simulink model "Quadcopter_ControllerWithNavigation"  (R2024b)
settings: Solver=FixedStepAuto  StartTime=0.0  StopTime=inf  RelTol=1e-3  EnableMultiTasking=on
undefined symbols (not defined in the file): SampleTime
libraries: px4uORBlib x10, slpidlib x10, simulink x4, uavalgslib x3, px4Utilslib x2, px4Peripheralslib x1, simulink_extras x1, sharedutil x1, sharedtransform x1
(part 1 of 3)
settings Model: ExtModeTrigDuration=10  Creator=The MathWorks, Inc.  LastModifiedBy=davi1
settings SolverCC: PositivePriorityOrder=on  MaxZcPerStep=1
settings OptimizationCC: EnhancedBackFolding=on  PassReuseOutputArgsAs=Individual arguments  ZeroExternalMemoryAtStartup=off  ZeroInternalMemoryAtStartup=off  MaxStackSize=64  OptimizeBlockOrder=speed  DifferentSizesBufferReuse=on  OptimizationCustomize=off  EfficientTunableParamExpr=on
settings DebuggingCC: ParameterTunabilityLossMsg=error
settings HardwareCC: ProdBitPerPointer=32  ProdBitPerSizeT=32  ProdBitPerPtrDiffT=32  ProdLargestAtomicInteger=Long  ProdLargestAtomicFloat=Double  ProdWordSize=32  ProdLongLongMode=on  ProdHWDeviceType=ARM Compatible->ARM Cortex
settings ModelReferenceCC: EnableRefExpFcnMdlSchedulingChecks=on
settings SFSimCC: MATLABDynamicMemAlloc=off  SimTargetLang=C++
settings RTWCC: Description=Embedded Coder  SystemTargetFile=ert.tlc  HardwareBoard=PX4 Pixhawk 6x  TLCOptions="-aInlineSetEventsForThisBaseRateFcn=TLC_FALSE -aSuppressMultiTaskScheduler=TLC_FALSE  -aRateBasedStepFcn=0"  TemplateMakefile=ert_default_tmf  Toolchain=GNU Tools for PX4 Autopilots  TargetLang=C++  GPUComputeCapability=3.5  DLArmComputeVersion=19.05
settings CodeAppCC: ForceParamTrailComments=on  IgnoreCustomStorageClasses=off  MaxIdLength=63  OperatorAnnotations=on  SimulinkDataObjDesc=on  SFDataObjDesc=on  InsertBlockDesc=on
settings ERTTargetCC: ExtModeTransport=3  ExtModeStaticAlloc=on  ExtModeStaticAllocSize=1024  ExtModeMexFile=ext_xcp  ExtModeIntrfLevel=Level2 - Open  InlinedParameterPlacement=Hierarchical

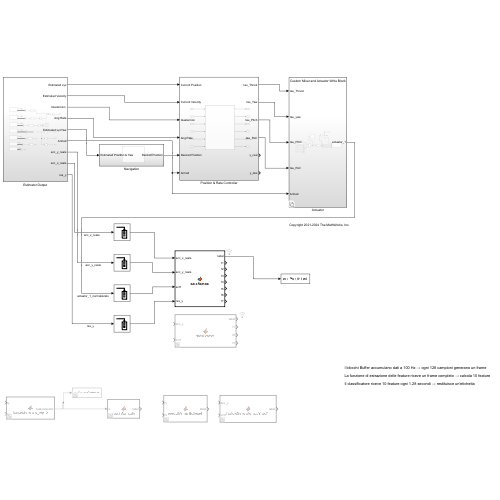
[thumbnail: Simulink's stored preview of the top-level diagram]
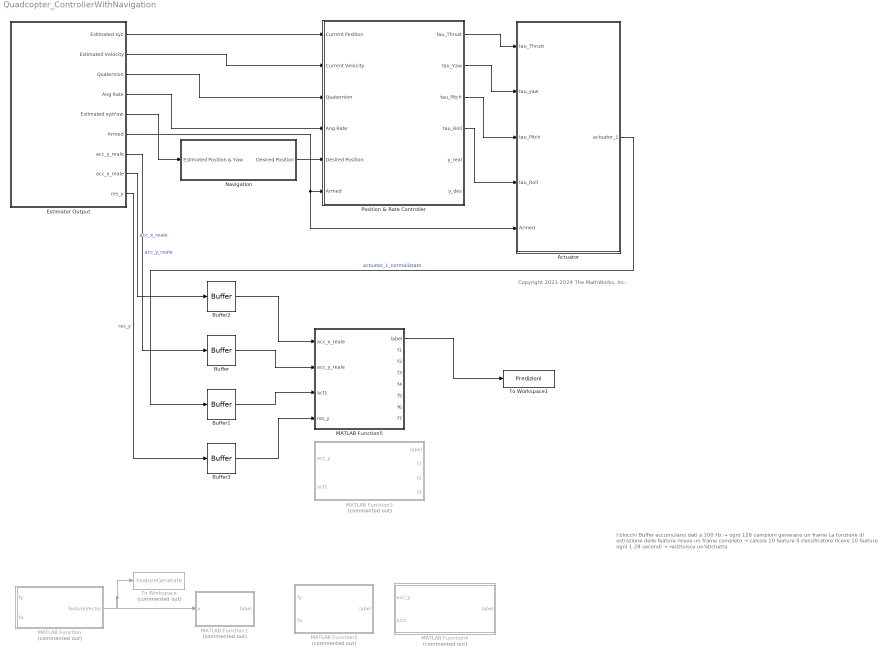
== system Quadcopter_ControllerWithNavigation ==
  note: I blocchi Buffer accumulano dati a 100 Hz → ogni 128 campioni generano un frame
      | La funzione di estrazione delle feature riceve un frame completo → calcola 10 feature
      | Il classificatore riceve 10 feature ogni 1.28 secondi → restituisce un'etichetta
  note: Copyright 2021-2024 The MathWorks, Inc.
  Actuator : Subsystem  Variant=on
  Buffer{,1..3} (4 alike) : Buffer  N=128  V=32  OutputFrames=off
  Estimator Output : Subsystem
  MATLAB Function : MATLAB Function  Commented=on  TreatAsAtomicUnit=on
  MATLAB Function1 : MATLAB Function  Commented=on  TreatAsAtomicUnit=on
  MATLAB Function2 : MATLAB Function  Commented=on  TreatAsAtomicUnit=on
  MATLAB Function3 : MATLAB Function  Commented=on  TreatAsAtomicUnit=on
  MATLAB Function4 : MATLAB Function  Commented=on  TreatAsAtomicUnit=on
  MATLAB Function5 : MATLAB Function  TreatAsAtomicUnit=on
  Navigation : Subsystem
  Position & Rate Controller : Subsystem
  To Workspace : ToWorkspace  Commented=on  VariableName=FeatureGenerate  SampleTime=-1
  To Workspace1 : ToWorkspace  VariableName=Predizioni  SaveFormat=Structure With Time  SampleTime=-1
  wires:
  Estimator Output/1(Estimated xyz) -> Position & Rate Controller/1(Current Position)
  Estimator Output/2(Estimated Velocity) -> Position & Rate Controller/2(Current Velocity)
  Estimator Output/3("Quaternion ") -> Position & Rate Controller/3(Quaternion)
  Navigation/1(Desired Position) -> Position & Rate Controller/5(Desired Position)
  Estimator Output/5(Estimated xyzYaw) -> Navigation/1(Estimated Position & Yaw)
  Estimator Output/4(Ang Rate) -> Position & Rate Controller/4(Ang Rate)
  Estimator Output/6(Armed) -> Actuator/5(Armed), Position & Rate Controller/6(Armed)
  Position & Rate Controller/1(tau_Thrust) -> Actuator/1(tau_Thrust)
  Position & Rate Controller/2(tau_Yaw) -> Actuator/2(tau_yaw)
  Position & Rate Controller/3(tau_Pitch) -> Actuator/3(tau_Pitch)
  Position & Rate Controller/4("tau_Roll ") -> Actuator/4(tau_Roll)
  MATLAB Function/1(featureVector) -> MATLAB Function1/1(x), To Workspace/1
  Estimator Output/7(acc_y_reale) -> Buffer/1  "acc_y_reale"
  Actuator/1(actuator_1) -> Buffer1/1  "actuator_1_normalizzato"
  Estimator Output/8(acc_x_reale) -> Buffer2/1  "acc_x_reale"
  Estimator Output/9(res_y) -> Buffer3/1  "res_y"
  Buffer2/1 -> MATLAB Function5/1(acc_x_reale)
  Buffer3/1 -> MATLAB Function5/4(res_y)
  Buffer/1 -> MATLAB Function5/2(acc_y_reale)
  Buffer1/1 -> MATLAB Function5/3(act1)
  MATLAB Function5/1(label) -> To Workspace1/1

== system Quadcopter_ControllerWithNavigation/Actuator ==
  tau_Thrust : Inport
  tau_yaw : Inport  Port=2
  tau_Pitch : Inport  Port=3
  tau_Roll : Inport  Port=4
  Armed : Inport  Port=5
  Custom Mixer and Actuator Write Block : Subsystem  VariantControl=useCustomMixer == true
  PX4 Mixer and actuator_controls_0 topic : Subsystem  VariantControl=useCustomMixer == false
  actuator_1 : Outport

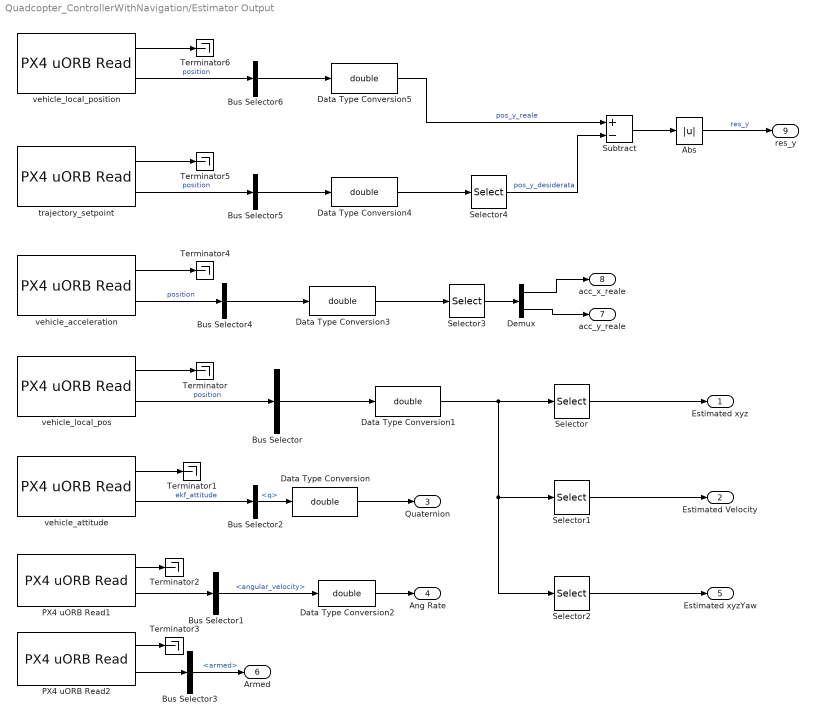
== system Quadcopter_ControllerWithNavigation/Estimator Output ==
  Abs : Abs  SaturateOnIntegerOverflow=off
  Bus Selector : BusSelector  OutputSignals=x,y,z,vx,vy,vz,heading  OutputAsBus=on
  Bus Selector1 : BusSelector  OutputSignals=angular_velocity
  Bus Selector2 : BusSelector  OutputSignals=q
  Bus Selector3 : BusSelector  OutputSignals=armed
  Bus Selector4 : BusSelector  OutputSignals=xyz  OutputAsBus=on
  Bus Selector5 : BusSelector  OutputSignals=position  OutputAsBus=on
  Bus Selector6 : BusSelector  OutputSignals=y  OutputAsBus=on
  Data Type Conversion{,1..5} (6 alike) : DataTypeConversion  OutDataTypeStr=double  SaturateOnIntegerOverflow=off  RndMeth=Floor
  Demux : Demux  Outputs=2
  PX4 uORB Read1 : px4uORBlib/PX4 uORB Read  uORBTopic=VehicleOdometry  selectInstance=vehicle_odometry  SampleTime=-1  BlockingMode=off  BlockTimeout=1e-3
  PX4 uORB Read2 : px4uORBlib/PX4 uORB Read  uORBTopic=ActuatorArmed  selectInstance=ActuatorArmed  SampleTime=-1  BlockingMode=off  BlockTimeout=1e-3
  Selector : Selector  InputPortWidth=7  IndexOptions=Index vector (dialog)  Indices=[1:3]  OutputSizes=1
  Selector1 : Selector  InputPortWidth=7  IndexOptions=Index vector (dialog)  Indices=[4:6]  OutputSizes=1
  Selector2 : Selector  InputPortWidth=7  IndexOptions=Index vector (dialog)  Indices=[1 2 3 7]  OutputSizes=1
  Selector3 : Selector  InputPortWidth=3  IndexOptions=Index vector (dialog)  Indices=[1 2]  OutputSizes=1
  Selector4 : Selector  InputPortWidth=3  IndexOptions=Index vector (dialog)  Indices=[2]  OutputSizes=1
  Subtract : Sum  Inputs=+-
  Terminator{,1..6} (7 alike) : Terminator
  trajectory_setpoint : px4uORBlib/PX4 uORB Read  uORBTopic=TrajectorySetpoint  selectInstance=TrajectorySetpoint  SampleTime=SampleTime  BlockingMode=off  BlockTimeout=1e-3
  vehicle_acceleration : px4uORBlib/PX4 uORB Read  uORBTopic=VehicleAcceleration  selectInstance=VehicleAcceleration  SampleTime=SampleTime  BlockingMode=off  BlockTimeout=1e-3
  vehicle_attitude : px4uORBlib/PX4 uORB Read  uORBTopic=VehicleAttitude  selectInstance=vehicle_attitude  SampleTime=-1  BlockingMode=off  BlockTimeout=1e-3
  vehicle_local_pos : px4uORBlib/PX4 uORB Read  uORBTopic=VehicleLocalPosition  selectInstance=vehicle_local_position  SampleTime=SampleTime  BlockingMode=off  BlockTimeout=1e-3
  vehicle_local_position : px4uORBlib/PX4 uORB Read  uORBTopic=VehicleLocalPosition  selectInstance=vehicle_local_position  SampleTime=SampleTime  BlockingMode=off  BlockTimeout=1e-3
  Estimated xyz : Outport
  Estimated Velocity : Outport  Port=2
  "Quaternion " : Outport  Port=3
  Ang Rate : Outport  Port=4
  Estimated xyzYaw : Outport  Port=5
  Armed : Outport  Port=6
  acc_y_reale : Outport  Port=7
  acc_x_reale : Outport  Port=8
  res_y : Outport  Port=9
  wires:
  Data Type Conversion/1 -> "Quaternion "/1
  Bus Selector2/1 -> Data Type Conversion/1  "<q>"
  vehicle_local_pos/2 -> Bus Selector/1  "position"
  Data Type Conversion1/1 -> Selector1/1, Selector2/1, Selector/1
  Selector2/1 -> Estimated xyzYaw/1
  vehicle_attitude/1 -> Terminator1/1
  vehicle_attitude/2 -> Bus Selector2/1  "ekf_attitude"
  vehicle_local_pos/1 -> Terminator/1
  Selector/1 -> Estimated xyz/1
  Selector1/1 -> Estimated Velocity/1
  Bus Selector/1 -> Data Type Conversion1/1
  PX4 uORB Read1/1 -> Terminator2/1
  Data Type Conversion2/1 -> Ang Rate/1
  PX4 uORB Read1/2 -> Bus Selector1/1
  PX4 uORB Read2/1 -> Terminator3/1
  Bus Selector3/1 -> Armed/1  "<armed>"
  PX4 uORB Read2/2 -> Bus Selector3/1
  Bus Selector1/1 -> Data Type Conversion2/1  "<angular_velocity>"
  vehicle_acceleration/1 -> Terminator4/1
  vehicle_acceleration/2 -> Bus Selector4/1  "position"
  Bus Selector4/1 -> Data Type Conversion3/1
  Data Type Conversion3/1 -> Selector3/1
  Bus Selector5/1 -> Data Type Conversion4/1
  trajectory_setpoint/2 -> Bus Selector5/1  "position"
  trajectory_setpoint/1 -> Terminator5/1
  Data Type Conversion4/1 -> Selector4/1
  Selector3/1 -> Demux/1
  Demux/2 -> acc_y_reale/1
  Demux/1 -> acc_x_reale/1
  vehicle_local_position/1 -> Terminator6/1
  Data Type Conversion5/1 -> Subtract/1  "pos_y_reale"
  vehicle_local_position/2 -> Bus Selector6/1  "position"
  Bus Selector6/1 -> Data Type Conversion5/1
  Selector4/1 -> Subtract/2  "pos_y_desiderata"
  Subtract/1 -> Abs/1
  Abs/1 -> res_y/1  "res_y"

== system Quadcopter_ControllerWithNavigation/Navigation ==
  Estimated Position & Yaw : Inport
  Quadcopter Navigation Algorithm : Subsystem  Variant=on
  Desired Position : Outport
  wires:
  Quadcopter Navigation Algorithm/1(Desired Position) -> Desired Position/1
  Estimated Position & Yaw/1 -> Quadcopter Navigation Algorithm/1(Current Position)

== system Quadcopter_ControllerWithNavigation/Position & Rate Controller ==
  Current Position : Inport
  Current Velocity : Inport  Port=2
  Quaternion : Inport  Port=3
  Ang Rate : Inport  Port=4
  Desired Position : Inport  Port=5
  Armed : Inport  Port=6
  Controller : Subsystem
  tau_Thrust : Outport
  tau_Yaw : Outport  Port=2
  tau_Pitch : Outport  Port=3
  "tau_Roll " : Outport  Port=4
  y_real : Outport  Port=5
  y_des : Outport  Port=6
  wires:
  Controller/3(tau_Pitch) -> tau_Pitch/1
  Quaternion/1 -> Controller/3(Quaternion)
  Controller/2(tau_Yaw) -> tau_Yaw/1
  Controller/4("tau_Roll ") -> "tau_Roll "/1
  Current Velocity/1 -> Controller/2(Velocity)
  Current Position/1 -> Controller/1(Position)
  Controller/1(tau_Thrust) -> tau_Thrust/1
  Desired Position/1 -> Controller/5(Desired Position)
  Ang Rate/1 -> Controller/4(Ang rate)
  Armed/1 -> Controller/6(Armed)
  Controller/5(y_real) -> y_real/1
  Controller/6(y_des) -> y_des/1

== system Quadcopter_ControllerWithNavigation/Actuator/Custom Mixer and Actuator Write Block ==
  tau_Thrust : Inport
  tau_yaw : Inport  Port=2
  tau_Pitch : Inport  Port=3
  tau_Roll : Inport  Port=4
  Armed : Inport  Port=5
  Data Type Conversion : DataTypeConversion  OutDataTypeStr=single  SaturateOnIntegerOverflow=off  RndMeth=Floor
  Demux : Demux
  Display : Display
  Mixer matrix : Constant  Value=[1 1 -1 1;1 -1 1 1;1 1 1 -1;1 -1 -1 -1]  OutDataTypeStr=Inherit: Inherit via back propagation  SampleTime=-1
  Mux1 : Mux
  PX4 Actuator Write : px4Peripheralslib/PX4 Actuator Write  Motor1Enable=on  Motor2Enable=on  Motor3Enable=on  Motor4Enable=on  Motor5Enable=off  Motor6Enable=off  Motor7Enable=off  Motor8Enable=off  Motor9Enable=off  Motor10Enable=off  Motor11Enable=off  Motor12Enable=off  IsMotorArray=off  Servo1Enable=off  Servo2Enable=off  Servo3Enable=off  Servo4Enable=off  Servo5Enable=off  Servo6Enable=off  Servo7Enable=off  Servo8Enable=off  IsServoArray=off
  Product1 : Product  Multiplication=Matrix(*)  RndMeth=Zero
  Saturation : Saturate  UpperLimit=1  LowerLimit=0
  Selector : Selector  InputPortWidth=4  IndexOptions=Index vector (dialog)  Indices=[1]  OutputSizes=1
  To Workspace : ToWorkspace  VariableName=Actuator1  SampleTime=-1
  actuator_1 : Outport
  wires:
  Demux/1 -> PX4 Actuator Write/2
  Demux/2 -> PX4 Actuator Write/3
  Product1/1 -> Display/1, Saturation/1
  Mux1/1 -> Product1/2
  Mixer matrix/1 -> Product1/1
  tau_yaw/1 -> Mux1/4
  tau_Thrust/1 -> Mux1/1  "thrust cmd"
  Saturation/1 -> Data Type Conversion/1
  tau_Roll/1 -> Mux1/3  "roll_cmd"
  Demux/3 -> PX4 Actuator Write/4
  Armed/1 -> PX4 Actuator Write/1
  tau_Pitch/1 -> Mux1/2  "pitch cmd"
  Demux/4 -> PX4 Actuator Write/5
  Data Type Conversion/1 -> Selector/1, Demux/1
  Selector/1 -> To Workspace/1, actuator_1/1

== system Quadcopter_ControllerWithNavigation/Actuator/PX4 Mixer and actuator_controls_0 topic ==
  tau_Thrust : Inport
  tau_yaw : Inport  Port=2
  tau_Pitch : Inport  Port=3
  tau_Roll : Inport  Port=4
  Armed : Inport  Port=5
  Bus Assignment : BusAssignment  AssignedSignals=control
  Constant : Constant  Value=zeros(4,1)
  Data Type Conversion : DataTypeConversion  SaturateOnIntegerOverflow=off  RndMeth=Floor
  Mux : Mux  Inputs=5
  PX4 uORB Message : px4uORBlib/PX4 uORB Message  uORBTopic=actuator_controls  SampleTime=inf  selectInstance=vehicle_gps_position
  PX4 uORB Write : px4uORBlib/PX4 uORB Write  uORBTopic=actuator_controls  selectInstance=actuator_controls_0  MessageQueueLen=1
  Terminator : Terminator
  wires:
  Bus Assignment/1 -> PX4 uORB Write/1
  tau_yaw/1 -> Mux/3
  Data Type Conversion/1 -> Bus Assignment/2
  tau_Roll/1 -> Mux/1  "roll_cmd"
  PX4 uORB Message/1 -> Bus Assignment/1
  Mux/1 -> Data Type Conversion/1
  Constant/1 -> Mux/5
  tau_Pitch/1 -> Mux/2  "pitch cmd"
  tau_Thrust/1 -> Mux/4  "thrust cmd"
  Armed/1 -> Terminator/1

== system Quadcopter_ControllerWithNavigation/Navigation/Quadcopter Navigation Algorithm ==
  Current Position : Inport
  Manual Waypoints : Subsystem  VariantControl=guidanceType == 3
  Manual Waypoints from Simulink Dashboard : Subsystem  VariantControl=guidanceType == 2
  Path Correction from Onboard Computer : Subsystem  VariantControl=guidanceType == 1
  Read waypoint from QGroundControl Mission : Subsystem  VariantControl=guidanceType == 0
  Desired Position : Outport

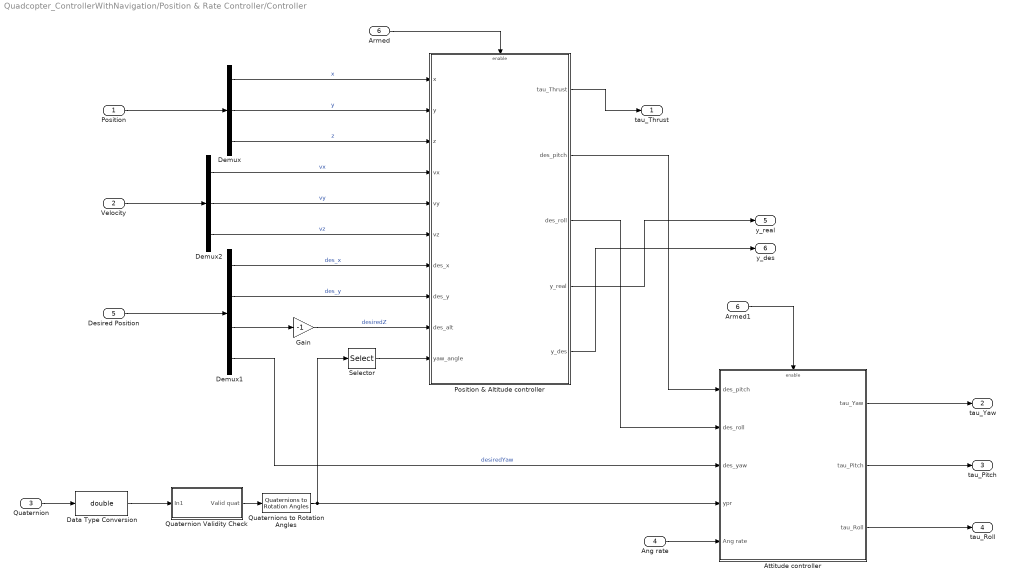
== system Quadcopter_ControllerWithNavigation/Position & Rate Controller/Controller ==
  Position : Inport
  Velocity : Inport  Port=2
  Quaternion : Inport  Port=3
  Ang rate : Inport  Port=4
  Desired Position : Inport  Port=5
  Armed : Inport  Port=6
  Armed1 : InportShadow  Port=6
  Attitude controller : Subsystem
  Data Type Conversion : DataTypeConversion  OutDataTypeStr=double  SaturateOnIntegerOverflow=off  RndMeth=Floor
  Demux : Demux  Outputs=3
  Demux1 : Demux
  Demux2 : Demux  Outputs=3
  Gain : Gain  Gain=-1
  Position & Altitude controller : Subsystem
  Quaternion Validity Check : Subsystem
  Quaternions to Rotation Angles : sharedtransform/Quaternions to Rotation Angles  rotationOrder=ZYX  aMode=aMode
  Selector : Selector  InputPortWidth=3  IndexOptions=Index vector (dialog)  Indices=[1]  OutputSizes=1
  tau_Thrust : Outport
  tau_Yaw : Outport  Port=2
  tau_Pitch : Outport  Port=3
  "tau_Roll " : Outport  Port=4
  y_real : Outport  Port=5
  y_des : Outport  Port=6
  wires:
  Attitude controller/3(tau_Roll) -> "tau_Roll "/1
  Attitude controller/2(tau_Pitch) -> tau_Pitch/1
  Attitude controller/1(tau_Yaw) -> tau_Yaw/1
  Position & Altitude controller/2(des_pitch) -> Attitude controller/1(des_pitch)
  Position & Altitude controller/3(des_roll) -> Attitude controller/2(des_roll)
  Demux/2 -> Position & Altitude controller/2(y)  "y"
  Gain/1 -> Position & Altitude controller/9(des_alt)  "desiredZ"
  Demux2/2 -> Position & Altitude controller/5(vy)  "vy"
  Demux1/1 -> Position & Altitude controller/7(des_x)  "des_x"
  Demux2/1 -> Position & Altitude controller/4(vx)  "vx"
  Demux1/3 -> Gain/1
  Demux/1 -> Position & Altitude controller/1(x)  "x"
  Demux1/2 -> Position & Altitude controller/8(des_y)  "des_y"
  Position & Altitude controller/1(tau_Thrust) -> tau_Thrust/1
  Desired Position/1 -> Demux1/1
  Demux2/3 -> Position & Altitude controller/6(vz)  "vz"
  Demux/3 -> Position & Altitude controller/3(z)  "z"
  Quaternion/1 -> Data Type Conversion/1
  Data Type Conversion/1 -> Quaternion Validity Check/1(In1)
  Position/1 -> Demux/1
  Velocity/1 -> Demux2/1
  Quaternion Validity Check/1(Valid quat) -> Quaternions to Rotation Angles/1
  Ang rate/1 -> Attitude controller/5(Ang rate)
  Quaternions to Rotation Angles/1 -> Selector/1, Attitude controller/4(ypr)
  Selector/1 -> Position & Altitude controller/10(yaw_angle)
  Demux1/4 -> Attitude controller/3(des_yaw)  "desiredYaw"
  Armed/1 -> Position & Altitude controller/Enable
  Armed1/1 -> Attitude controller/Enable
  Position & Altitude controller/4(y_real) -> y_real/1
  Position & Altitude controller/5(y_des) -> y_des/1

== system Quadcopter_ControllerWithNavigation/Navigation/Quadcopter Navigation Algorithm/Manual Waypoints ==
  Current Position : Inport
  Constant1 : Constant  Value=[0 0 -20 0; 20 0 -20 0;20 10 -20 0; 20 100 -30 0;30 100 -30 0;50 100 -30 0]  SampleTime=-1
  Constant2 : Constant  Value=2  SampleTime=-1
  Constant3 : Constant  Value=0  SampleTime=-1
  Mux : Mux  Inputs=2
  Subsystem : Subsystem
  Switch : Switch  Criteria=u2 > Threshold  SaturateOnIntegerOverflow=off  InputSameDT=off
  Terminator1 : Terminator
  Terminator2 : Terminator
  Terminator4 : Terminator
  Waypoint Follower : uavalgslib/Waypoint Follower  UAVType=multirotor  StartFrom=first  TransitionRadiusSource=internal  TransitionRadius=5  MinLookaheadDistance=0.1  HoverAtLastWaypoint=off  YawInput=on  ShowCrossTrackErrorOutput=off  ShowStatusOutput=on  SimulateUsing=Interpreted execution
  Desired Position : Outport
  wires:
  Constant1/1 -> Waypoint Follower/2
  Waypoint Follower/1 -> Subsystem/2(Lookahead Point), Switch/3
  Waypoint Follower/4 -> Terminator4/1
  Subsystem/1(des_landing_pos) -> Switch/1
  Current Position/1 -> Waypoint Follower/1, Subsystem/1(curr_xyzYaw)
  Waypoint Follower/5 -> Switch/2
  Constant2/1 -> Waypoint Follower/3
  Waypoint Follower/2 -> Terminator2/1
  Switch/1 -> Mux/1  "command"
  Mux/1 -> Desired Position/1
  Waypoint Follower/3 -> Terminator1/1
  Constant3/1 -> Mux/2

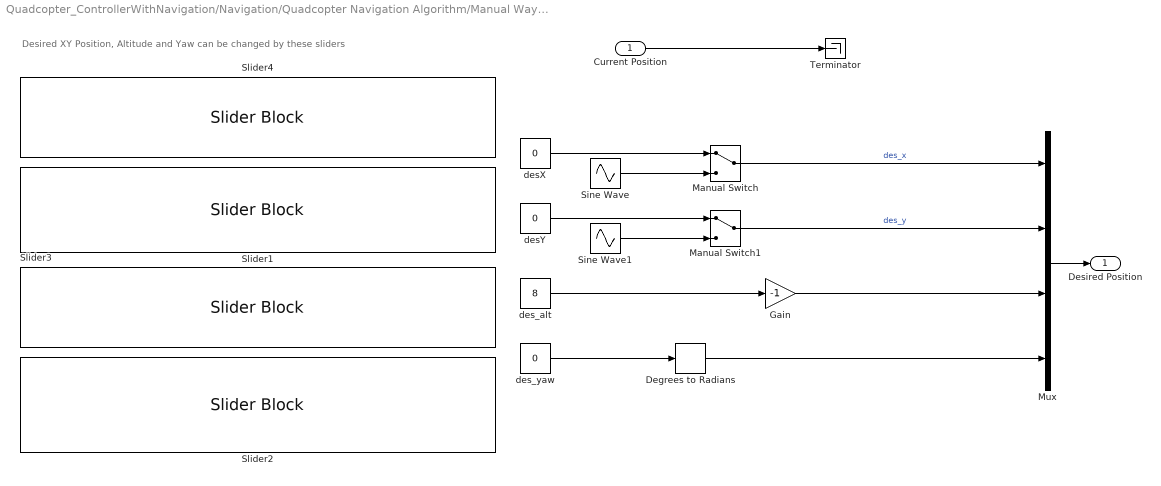
== system Quadcopter_ControllerWithNavigation/Navigation/Quadcopter Navigation Algorithm/Manual Waypoints from Simulink Dashboard ==
  note: Desired XY Position, Altitude and Yaw can be changed by these sliders
  Current Position : Inport  PortDimensions=[1 4]
  Degrees to Radians : simulink_extras/Transformations/Degrees to Radians
  Gain : Gain  Gain=-1
  Manual Switch : ManualSwitch
  Manual Switch1 : ManualSwitch
  Mux : Mux
  Sine Wave : Sin  Amplitude=80  Frequency=2*pi*0.005
  Sine Wave1 : Sin  Amplitude=80  Frequency=2*pi*0.005  Phase=pi/2
  Slider1 : SliderBlock  ScaleMin=-20  ScaleMax=20
  Slider2 : SliderBlock  ScaleMin=-180  ScaleMax=180
  Slider3 : SliderBlock
  Slider4 : SliderBlock  ScaleMin=-20  ScaleMax=20
  Terminator : Terminator
  desX : Constant  Value=0  SampleTime=-1
  desY : Constant  Value=0  SampleTime=-1
  des_alt : Constant  Value=8  SampleTime=-1
  des_yaw : Constant  Value=0  SampleTime=-1
  Desired Position : Outport
  wires:
  des_alt/1 -> Gain/1
  desY/1 -> Manual Switch1/1
  Sine Wave/1 -> Manual Switch/2
  desX/1 -> Manual Switch/1
  Manual Switch1/1 -> Mux/2  "des_y"
  des_yaw/1 -> Degrees to Radians/1
  Manual Switch/1 -> Mux/1  "des_x"
  Sine Wave1/1 -> Manual Switch1/2
  Mux/1 -> Desired Position/1
  Current Position/1 -> Terminator/1
  Gain/1 -> Mux/3
  Degrees to Radians/1 -> Mux/4

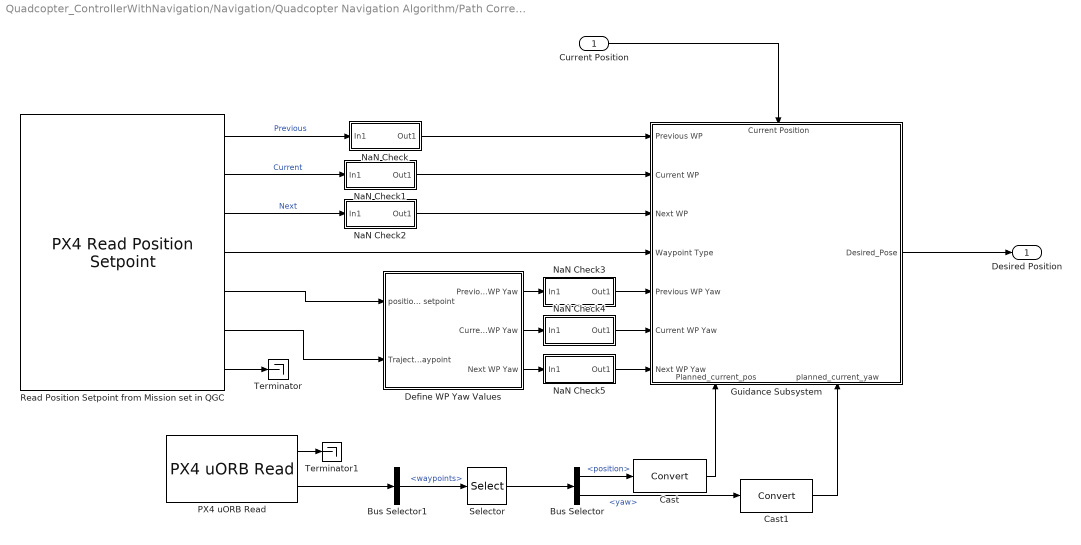
== system Quadcopter_ControllerWithNavigation/Navigation/Quadcopter Navigation Algorithm/Path Correction from Onboard Computer ==
  Current Position : Inport
  Bus Selector : BusSelector  OutputSignals=position,yaw
  Bus Selector1 : BusSelector  OutputSignals=waypoints
  Cast : DataTypeConversion  SaturateOnIntegerOverflow=off  RndMeth=Floor
  Cast1 : DataTypeConversion  SaturateOnIntegerOverflow=off  RndMeth=Floor
  "Define WP Yaw Values " : Subsystem
  Guidance Subsystem : Subsystem
      settings: PortSchema="{\"entries\":[{\"content\":{\"sides\":[{\"content\":{\"connectorIds\":[\"In1\",\"In2\",\"In3\",\"In4\",\"In5\",\"In6\",\"In7\"]},\"type\":\"ConnectorPlacement.EquallySpacedRectSide\",\"uuid\":\"e9e96be5-af21-4911-860e-f3d41d3d51a5\"},{\"content\":{\"connectorIds\":[\"Out1\"],\"side\":\"RIGHT\"},\"type\":\"ConnectorPlacement.EquallySpacedRectSide\",\"uuid\":\"1d190cc4-2348-4eca-a529-c9f1d728b718\"},{\"content\":{\"connectorIds\":[\"In8\"],\"side\":\"TOP\"},\"type\":\"ConnectorPlacement.EquallySpacedRectSide\",\"uuid\":\"c248d3d5-3b30-416c-a277-519f6ee966ff\"},{\"content\":{\"connectorIds\":[\"In9\",\"In10\"],\"side\":\"BOTTOM\"},\"type\":\"ConnectorPlacement.EquallySpacedRectSide\",\"uuid\":\"2b8da87f-17bd-449d-af9e-128c1548c7b5\"}]},\"type\":\"ConnectorPlacement.EquallySpacedConnector\",\"uuid\":\"bbf0c511-85fc-440a-b356-10e645af4727\"}],\"packageUris\":[\"http://schema.mathworks.com/mf0/Connector/R2020b\"],\"version\":\"1.0\"}"
  NaN Check : Subsystem
  NaN Check1 : Subsystem
  NaN Check2 : Subsystem
  NaN Check3 : Subsystem
  NaN Check4 : Subsystem
  NaN Check5 : Subsystem
  PX4 uORB Read : px4uORBlib/PX4 uORB Read  uORBTopic=vehicle_trajectory_waypoint  selectInstance=vehicle_trajectory_waypoint_desired  SampleTime=SampleTime  BlockingMode=off  BlockTimeout=1e-3
  Read Position Setpoint from Mission set in QGC : px4Utilslib/PX4 Read Position Setpoint  coordinateFrame=Local Coordinates (NED)  SampleTime=SampleTime  positionSetpointBus=on  trajectoryWaypointsBus=on  onboardFailsafeFlag=off  onboardEnableStatus=on
  Selector : Selector  InputPortWidth=5  IndexOptions=Index vector (dialog)  Indices=2  OutputSizes=1
  Terminator : Terminator
  Terminator1 : Terminator
  Desired Position : Outport
  wires:
  Read Position Setpoint from Mission set in QGC/2 -> NaN Check1/1(In1)  "Current"
  Read Position Setpoint from Mission set in QGC/4 -> Guidance Subsystem/4(Waypoint Type)
  Read Position Setpoint from Mission set in QGC/1 -> NaN Check/1(In1)  "Previous"
  Guidance Subsystem/1(Desired_Pose) -> Desired Position/1
  Read Position Setpoint from Mission set in QGC/3 -> NaN Check2/1(In1)  "Next"
  Current Position/1 -> Guidance Subsystem/8(Current Position)
  Read Position Setpoint from Mission set in QGC/7 -> Terminator/1
  Read Position Setpoint from Mission set in QGC/6 -> "Define WP Yaw Values "/2(Trajectory Waypoint)
  Read Position Setpoint from Mission set in QGC/5 -> "Define WP Yaw Values "/1(position setpoint)
  "Define WP Yaw Values "/3(Next WP Yaw) -> NaN Check5/1(In1)
  "Define WP Yaw Values "/2(Current WP Yaw) -> NaN Check4/1(In1)
  "Define WP Yaw Values "/1(Previous WP Yaw) -> NaN Check3/1(In1)
  PX4 uORB Read/1 -> Terminator1/1
  Bus Selector/1 -> Cast/1  "<position>"
  PX4 uORB Read/2 -> Bus Selector1/1
  Selector/1 -> Bus Selector/1
  Bus Selector/2 -> Cast1/1  "<yaw>"
  Bus Selector1/1 -> Selector/1  "<waypoints>"
  Cast/1 -> Guidance Subsystem/9(Planned_current_pos)
  Cast1/1 -> Guidance Subsystem/10(planned_current_yaw)
  NaN Check/1(Out1) -> Guidance Subsystem/1(Previous WP)
  NaN Check1/1(Out1) -> Guidance Subsystem/2(Current WP)
  NaN Check2/1(Out1) -> Guidance Subsystem/3(Next WP)
  NaN Check3/1(Out1) -> Guidance Subsystem/5(Previous WP Yaw)
  NaN Check4/1(Out1) -> Guidance Subsystem/6(Current WP Yaw)
  NaN Check5/1(Out1) -> Guidance Subsystem/7(Next WP Yaw)

== system Quadcopter_ControllerWithNavigation/Navigation/Quadcopter Navigation Algorithm/Read waypoint from QGroundControl Mission ==
  Current Position : Inport
  Guidance Subsystem : Subsystem
      settings: PortSchema="{\"entries\":[{\"content\":{\"sides\":[{\"content\":{\"connectorIds\":[\"In1\",\"In2\",\"In3\",\"In4\"]},\"type\":\"ConnectorPlacement.EquallySpacedRectSide\",\"uuid\":\"e9e96be5-af21-4911-860e-f3d41d3d51a5\"},{\"content\":{\"connectorIds\":[\"Out1\"],\"side\":\"RIGHT\"},\"type\":\"ConnectorPlacement.EquallySpacedRectSide\",\"uuid\":\"1d190cc4-2348-4eca-a529-c9f1d728b718\"},{\"content\":{\"connectorIds\":[\"In5\"],\"side\":\"TOP\"},\"type\":\"ConnectorPlacement.EquallySpacedRectSide\",\"uuid\":\"c248d3d5-3b30-416c-a277-519f6ee966ff\"}]},\"type\":\"ConnectorPlacement.EquallySpacedConnector\",\"uuid\":\"bbf0c511-85fc-440a-b356-10e645af4727\"}],\"packageUris\":[\"http://schema.mathworks.com/mf0/Connector/R2020b\"],\"version\":\"1.0\"}"
  Read Position Setpoint from Mission set in QGC : px4Utilslib/PX4 Read Position Setpoint  coordinateFrame=Local Coordinates (NED)  SampleTime=SampleTime  positionSetpointBus=off  trajectoryWaypointsBus=off  onboardFailsafeFlag=off  onboardEnableStatus=off
  Desired Position : Outport
  wires:
  Read Position Setpoint from Mission set in QGC/1 -> Guidance Subsystem/1(Previous WP)  "Previous"
  Read Position Setpoint from Mission set in QGC/4 -> Guidance Subsystem/4(Waypoint Type)
  Read Position Setpoint from Mission set in QGC/2 -> Guidance Subsystem/2(Current WP)  "Current"
  Guidance Subsystem/1(Desired_Pose) -> Desired Position/1
  Read Position Setpoint from Mission set in QGC/3 -> Guidance Subsystem/3(Next WP)  "Next"
  Current Position/1 -> Guidance Subsystem/5(Current Position)

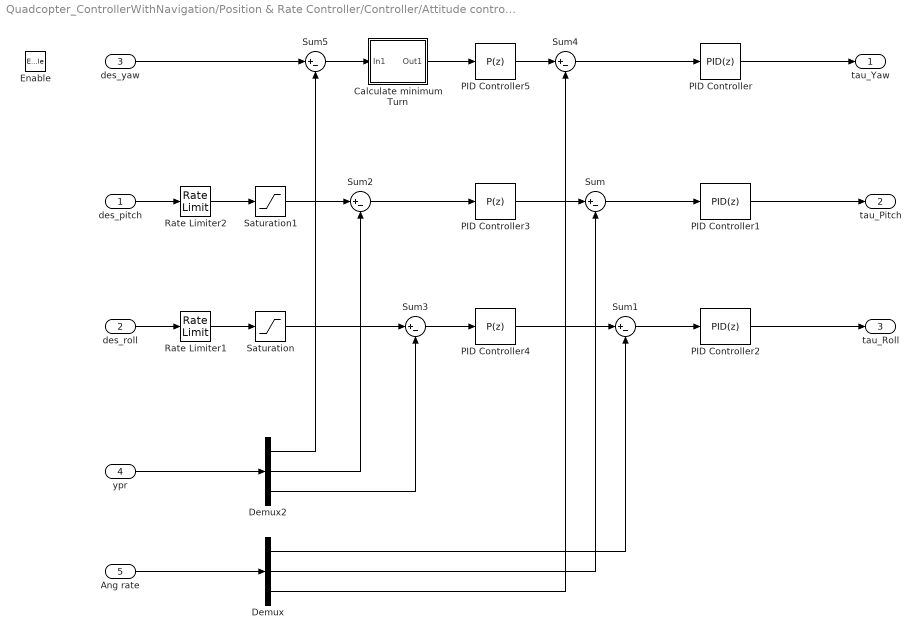
== system Quadcopter_ControllerWithNavigation/Position & Rate Controller/Controller/Attitude controller ==
  des_pitch : Inport
  des_roll : Inport  Port=2
  des_yaw : Inport  Port=3
  ypr : Inport  Port=4
  Ang rate : Inport  Port=5
  Enable : EnablePort
  Calculate minimum Turn : Subsystem
  Demux : Demux  Outputs=3
  Demux2 : Demux  Outputs=3
  PID Controller : slpidlib/PID Controller  Controller=PID  Form=Parallel  TimeDomain=Discrete-time  UseExternalTs=off  SampleTime=-1  IntegratorMethod=Forward Euler  FilterMethod=Forward Euler  ControllerParametersSource=internal  P=0.2  I=0  UseKiTs=off  D=0  UseExternalDerivativeSource=off  N=100  UseFilter=on  TunerSelectOption=Transfer Function Based (PID Tuner App)  InitialConditionSource=internal  InitialConditionForIntegrator=0  InitialConditionForFilter=0  DifferentiatorICPrevScaledInput=0  ExternalReset=none  TrackingMode=off  Kt=1  LimitOutput=on  SatLimitsSource=internal  UpperSaturationLimit=0.1  LowerSaturationLimit=-0.1  LinearizeAsGain=on  AntiWindupMode=clamping  Kb=1  LimitIntegrator=off  UpperIntegratorSaturationLimit=inf  LowerIntegratorSaturationLimit=-inf  POutMin=[]  POutMax=[]  IOutMin=[]  IOutMax=[]  DOutMin=[]  DOutMax=[]  NOutMin=[]  NOutMax=[]  SumOutMin=[]  SumOutMax=[]  SaturationOutMin=[]  SaturationOutMax=[]  PParamMin=[]  PParamMax=[]  IParamMin=[]  IParamMax=[]  DParamMin=[]  DParamMax=[]  NParamMin=[]  NParamMax=[]  KbParamMin=[]  KbParamMax=[]  KtParamMin=[]  KtParamMax=[]  KbOutMin=[]  KbOutMax=[]  KtOutMin=[]  KtOutMax=[]  IntegratorOutMin=[]  IntegratorOutMax=[]  FilterOutMin=[]  FilterOutMax=[]  SumI1OutMin=[]  SumI1OutMax=[]  SumI2OutMin=[]  SumI2OutMax=[]  SumI3OutMin=[]  SumI3OutMax=[]  SumI4OutMin=[]  SumI4OutMax=[]  SumDOutMin=[]  SumDOutMax=[]  DifferentiatorOutMin=[]  DifferentiatorOutMax=[]  FilterDiffOutCoefMin=[]  FilterDiffOutCoefMax=[]  ReciprocalOutMin=[]  ReciprocalOutMax=[]  SumDenOutMin=[]  SumDenOutMax=[]  SumNumOutMin=[]  SumNumOutMax=[]  DivideOutMin=[]  DivideOutMax=[]  UdiffTsProdOutMin=[]  UdiffTsProdOutMax=[]  NTsProdOutMin=[]  NTsProdOutMax=[]  UintegralTsProdOutMin=[]  UintegralTsProdOutMax=[]  UngainTsProdOutMin=[]  UngainTsProdOutMax=[]  ClampingZeroOutDataTypeStr=Inherit: Inherit via back propagation  ClampingZeroOutMin=[]  ClampingZeroOutMax=[]  FilterDenConstantOutDataTypeStr=Inherit: Inherit via back propagation  FilterDenConstantOutMin=[]  FilterDenConstantOutMax=[]  PCopyOutDataTypeStr=Inherit: Inherit via back propagation  PCopyOutMin=[]  PCopyOutMax=[]  NCopyOutDataTypeStr=Inherit: Inherit via back propagation  NCopyOutMin=[]  NCopyOutMax=[]  IntegratorContinuousStateAttributes=''  IntegratorStateMustResolveToSignalObject=off  IntegratorRTWStateStorageClass=Auto  FilterContinuousStateAttributes=''  FilterStateMustResolveToSignalObject=off  FilterRTWStateStorageClass=Auto  ParallelPVariant=InternalParameters  IdealPVariant=Disabled  IVariant=InternalParameters  DVariant=InternalParameters  IntegratorVariant=Discrete  SatVariant=Enabled  AWVariant=DiscClampingParallel  PCopyVariant=Disabled  TRVariant=Disabled  FdbkBlocksVariant=Forward  IdealPFdbkVariant=Disabled  SatFdbkVariant=Disabled  DerivativeFilterVariant=ForwardEulerFilter  NVariant=InternalParameters  NCopyVariant=Disabled  FilterICVariant=InternalICsFilter  IntegratorICVariant=InternalICs  ExternalResetVariant=Disabled  TRSumVariant=Passthrough  SumFdbkVariant=Disabled  SumVariant=Sum_PID  TsampFilterVariant=InternalTs  TsampNgainVariant=Passthrough  TsampIntegralVariant=Disabled_SignalSpec  ExternalSaturationOutDataTypeStr=Inherit: Same as second input  DerivativeSourceVariant=ErrorSignal  PreIntVariant=InternalPreInt
  PID Controller1 : slpidlib/PID Controller  Controller=PID  Form=Parallel  TimeDomain=Discrete-time  UseExternalTs=off  SampleTime=-1  IntegratorMethod=Forward Euler  FilterMethod=Forward Euler  ControllerParametersSource=internal  P=0.035  I=0  UseKiTs=off  D=0.05/20  UseExternalDerivativeSource=off  N=50  UseFilter=on  TunerSelectOption=Transfer Function Based (PID Tuner App)  InitialConditionSource=internal  InitialConditionForIntegrator=0  InitialConditionForFilter=0  DifferentiatorICPrevScaledInput=0  ExternalReset=none  TrackingMode=off  Kt=1  LimitOutput=on  SatLimitsSource=internal  UpperSaturationLimit=0.2  LowerSaturationLimit=-0.2  LinearizeAsGain=on  AntiWindupMode=clamping  Kb=1  LimitIntegrator=off  UpperIntegratorSaturationLimit=inf  LowerIntegratorSaturationLimit=-inf  POutMin=[]  POutMax=[]  IOutMin=[]  IOutMax=[]  DOutMin=[]  DOutMax=[]  NOutMin=[]  NOutMax=[]  SumOutMin=[]  SumOutMax=[]  SaturationOutMin=[]  SaturationOutMax=[]  PParamMin=[]  PParamMax=[]  IParamMin=[]  IParamMax=[]  DParamMin=[]  DParamMax=[]  NParamMin=[]  NParamMax=[]  KbParamMin=[]  KbParamMax=[]  KtParamMin=[]  KtParamMax=[]  KbOutMin=[]  KbOutMax=[]  KtOutMin=[]  KtOutMax=[]  IntegratorOutMin=[]  IntegratorOutMax=[]  FilterOutMin=[]  FilterOutMax=[]  SumI1OutMin=[]  SumI1OutMax=[]  SumI2OutMin=[]  SumI2OutMax=[]  SumI3OutMin=[]  SumI3OutMax=[]  SumI4OutMin=[]  SumI4OutMax=[]  SumDOutMin=[]  SumDOutMax=[]  DifferentiatorOutMin=[]  DifferentiatorOutMax=[]  FilterDiffOutCoefMin=[]  FilterDiffOutCoefMax=[]  ReciprocalOutMin=[]  ReciprocalOutMax=[]  SumDenOutMin=[]  SumDenOutMax=[]  SumNumOutMin=[]  SumNumOutMax=[]  DivideOutMin=[]  DivideOutMax=[]  UdiffTsProdOutMin=[]  UdiffTsProdOutMax=[]  NTsProdOutMin=[]  NTsProdOutMax=[]  UintegralTsProdOutMin=[]  UintegralTsProdOutMax=[]  UngainTsProdOutMin=[]  UngainTsProdOutMax=[]  ClampingZeroOutDataTypeStr=Inherit: Inherit via back propagation  ClampingZeroOutMin=[]  ClampingZeroOutMax=[]  FilterDenConstantOutDataTypeStr=Inherit: Inherit via back propagation  FilterDenConstantOutMin=[]  FilterDenConstantOutMax=[]  PCopyOutDataTypeStr=Inherit: Inherit via back propagation  PCopyOutMin=[]  PCopyOutMax=[]  NCopyOutDataTypeStr=Inherit: Inherit via back propagation  NCopyOutMin=[]  NCopyOutMax=[]  IntegratorContinuousStateAttributes=''  IntegratorStateMustResolveToSignalObject=off  IntegratorRTWStateStorageClass=Auto  FilterContinuousStateAttributes=''  FilterStateMustResolveToSignalObject=off  FilterRTWStateStorageClass=Auto  ParallelPVariant=InternalParameters  IdealPVariant=Disabled  IVariant=InternalParameters  DVariant=InternalParameters  IntegratorVariant=Discrete  SatVariant=Enabled  AWVariant=DiscClampingParallel  PCopyVariant=Disabled  TRVariant=Disabled  FdbkBlocksVariant=Forward  IdealPFdbkVariant=Disabled  SatFdbkVariant=Disabled  DerivativeFilterVariant=ForwardEulerFilter  NVariant=InternalParameters  NCopyVariant=Disabled  FilterICVariant=InternalICsFilter  IntegratorICVariant=InternalICs  ExternalResetVariant=Disabled  TRSumVariant=Passthrough  SumFdbkVariant=Disabled  SumVariant=Sum_PID  TsampFilterVariant=InternalTs  TsampNgainVariant=Passthrough  TsampIntegralVariant=Disabled_SignalSpec  ExternalSaturationOutDataTypeStr=Inherit: Same as second input  DerivativeSourceVariant=ErrorSignal  PreIntVariant=InternalPreInt
  PID Controller2 : slpidlib/PID Controller  Controller=PID  Form=Parallel  TimeDomain=Discrete-time  UseExternalTs=off  SampleTime=-1  IntegratorMethod=Forward Euler  FilterMethod=Forward Euler  ControllerParametersSource=internal  P=0.035  I=0  UseKiTs=off  D=0.05/20  UseExternalDerivativeSource=off  N=50  UseFilter=on  TunerSelectOption=Transfer Function Based (PID Tuner App)  InitialConditionSource=internal  InitialConditionForIntegrator=0  InitialConditionForFilter=0  DifferentiatorICPrevScaledInput=0  ExternalReset=none  TrackingMode=off  Kt=1  LimitOutput=on  SatLimitsSource=internal  UpperSaturationLimit=0.2  LowerSaturationLimit=-0.2  LinearizeAsGain=on  AntiWindupMode=clamping  Kb=1  LimitIntegrator=off  UpperIntegratorSaturationLimit=inf  LowerIntegratorSaturationLimit=-inf  POutMin=[]  POutMax=[]  IOutMin=[]  IOutMax=[]  DOutMin=[]  DOutMax=[]  NOutMin=[]  NOutMax=[]  SumOutMin=[]  SumOutMax=[]  SaturationOutMin=[]  SaturationOutMax=[]  PParamMin=[]  PParamMax=[]  IParamMin=[]  IParamMax=[]  DParamMin=[]  DParamMax=[]  NParamMin=[]  NParamMax=[]  KbParamMin=[]  KbParamMax=[]  KtParamMin=[]  KtParamMax=[]  KbOutMin=[]  KbOutMax=[]  KtOutMin=[]  KtOutMax=[]  IntegratorOutMin=[]  IntegratorOutMax=[]  FilterOutMin=[]  FilterOutMax=[]  SumI1OutMin=[]  SumI1OutMax=[]  SumI2OutMin=[]  SumI2OutMax=[]  SumI3OutMin=[]  SumI3OutMax=[]  SumI4OutMin=[]  SumI4OutMax=[]  SumDOutMin=[]  SumDOutMax=[]  DifferentiatorOutMin=[]  DifferentiatorOutMax=[]  FilterDiffOutCoefMin=[]  FilterDiffOutCoefMax=[]  ReciprocalOutMin=[]  ReciprocalOutMax=[]  SumDenOutMin=[]  SumDenOutMax=[]  SumNumOutMin=[]  SumNumOutMax=[]  DivideOutMin=[]  DivideOutMax=[]  UdiffTsProdOutMin=[]  UdiffTsProdOutMax=[]  NTsProdOutMin=[]  NTsProdOutMax=[]  UintegralTsProdOutMin=[]  UintegralTsProdOutMax=[]  UngainTsProdOutMin=[]  UngainTsProdOutMax=[]  ClampingZeroOutDataTypeStr=Inherit: Inherit via back propagation  ClampingZeroOutMin=[]  ClampingZeroOutMax=[]  FilterDenConstantOutDataTypeStr=Inherit: Inherit via back propagation  FilterDenConstantOutMin=[]  FilterDenConstantOutMax=[]  PCopyOutDataTypeStr=Inherit: Inherit via back propagation  PCopyOutMin=[]  PCopyOutMax=[]  NCopyOutDataTypeStr=Inherit: Inherit via back propagation  NCopyOutMin=[]  NCopyOutMax=[]  IntegratorContinuousStateAttributes=''  IntegratorStateMustResolveToSignalObject=off  IntegratorRTWStateStorageClass=Auto  FilterContinuousStateAttributes=''  FilterStateMustResolveToSignalObject=off  FilterRTWStateStorageClass=Auto  ParallelPVariant=InternalParameters  IdealPVariant=Disabled  IVariant=InternalParameters  DVariant=InternalParameters  IntegratorVariant=Discrete  SatVariant=Enabled  AWVariant=DiscClampingParallel  PCopyVariant=Disabled  TRVariant=Disabled  FdbkBlocksVariant=Forward  IdealPFdbkVariant=Disabled  SatFdbkVariant=Disabled  DerivativeFilterVariant=ForwardEulerFilter  NVariant=InternalParameters  NCopyVariant=Disabled  FilterICVariant=InternalICsFilter  IntegratorICVariant=InternalICs  ExternalResetVariant=Disabled  TRSumVariant=Passthrough  SumFdbkVariant=Disabled  SumVariant=Sum_PID  TsampFilterVariant=InternalTs  TsampNgainVariant=Passthrough  TsampIntegralVariant=Disabled_SignalSpec  ExternalSaturationOutDataTypeStr=Inherit: Same as second input  DerivativeSourceVariant=ErrorSignal  PreIntVariant=InternalPreInt
  PID Controller3 : slpidlib/PID Controller  Controller=P  Form=Parallel  TimeDomain=Discrete-time  UseExternalTs=off  SampleTime=-1  IntegratorMethod=Forward Euler  FilterMethod=Forward Euler  ControllerParametersSource=internal  P=4  I=1  UseKiTs=off  D=0  UseExternalDerivativeSource=off  N=100  UseFilter=on  TunerSelectOption=Transfer Function Based (PID Tuner App)  InitialConditionSource=internal  InitialConditionForIntegrator=0  InitialConditionForFilter=0  DifferentiatorICPrevScaledInput=0  ExternalReset=none  TrackingMode=off  Kt=1  LimitOutput=off  SatLimitsSource=internal  UpperSaturationLimit=inf  LowerSaturationLimit=-inf  LinearizeAsGain=on  AntiWindupMode=none  Kb=1  LimitIntegrator=off  UpperIntegratorSaturationLimit=inf  LowerIntegratorSaturationLimit=-inf  POutMin=[]  POutMax=[]  IOutMin=[]  IOutMax=[]  DOutMin=[]  DOutMax=[]  NOutMin=[]  NOutMax=[]  SumOutMin=[]  SumOutMax=[]  SaturationOutMin=[]  SaturationOutMax=[]  PParamMin=[]  PParamMax=[]  IParamMin=[]  IParamMax=[]  DParamMin=[]  DParamMax=[]  NParamMin=[]  NParamMax=[]  KbParamMin=[]  KbParamMax=[]  KtParamMin=[]  KtParamMax=[]  KbOutMin=[]  KbOutMax=[]  KtOutMin=[]  KtOutMax=[]  IntegratorOutMin=[]  IntegratorOutMax=[]  FilterOutMin=[]  FilterOutMax=[]  SumI1OutMin=[]  SumI1OutMax=[]  SumI2OutMin=[]  SumI2OutMax=[]  SumI3OutMin=[]  SumI3OutMax=[]  SumI4OutMin=[]  SumI4OutMax=[]  SumDOutMin=[]  SumDOutMax=[]  DifferentiatorOutMin=[]  DifferentiatorOutMax=[]  FilterDiffOutCoefMin=[]  FilterDiffOutCoefMax=[]  ReciprocalOutMin=[]  ReciprocalOutMax=[]  SumDenOutMin=[]  SumDenOutMax=[]  SumNumOutMin=[]  SumNumOutMax=[]  DivideOutMin=[]  DivideOutMax=[]  UdiffTsProdOutMin=[]  UdiffTsProdOutMax=[]  NTsProdOutMin=[]  NTsProdOutMax=[]  UintegralTsProdOutMin=[]  UintegralTsProdOutMax=[]  UngainTsProdOutMin=[]  UngainTsProdOutMax=[]  ClampingZeroOutDataTypeStr=Inherit: Inherit via back propagation  ClampingZeroOutMin=[]  ClampingZeroOutMax=[]  FilterDenConstantOutDataTypeStr=Inherit: Inherit via back propagation  FilterDenConstantOutMin=[]  FilterDenConstantOutMax=[]  PCopyOutDataTypeStr=Inherit: Inherit via back propagation  PCopyOutMin=[]  PCopyOutMax=[]  NCopyOutDataTypeStr=Inherit: Inherit via back propagation  NCopyOutMin=[]  NCopyOutMax=[]  IntegratorContinuousStateAttributes=''  IntegratorStateMustResolveToSignalObject=off  IntegratorRTWStateStorageClass=Auto  FilterContinuousStateAttributes=''  FilterStateMustResolveToSignalObject=off  FilterRTWStateStorageClass=Auto  ParallelPVariant=InternalParameters  IdealPVariant=Disabled  IVariant=Disabled  DVariant=Disabled  IntegratorVariant=Disabled  SatVariant=Disabled  AWVariant=Disabled  PCopyVariant=Disabled  TRVariant=Disabled  FdbkBlocksVariant=Forward  IdealPFdbkVariant=Disabled  SatFdbkVariant=Disabled  DerivativeFilterVariant=Disabled  NVariant=Disabled  NCopyVariant=Disabled_SignalSpec  FilterICVariant=Disabled  IntegratorICVariant=Disabled  ExternalResetVariant=Disabled  TRSumVariant=Passthrough  SumFdbkVariant=Disabled  SumVariant=Passthrough_P  TsampFilterVariant=InternalTs  TsampNgainVariant=Passthrough  TsampIntegralVariant=Disabled_SignalSpec  ExternalSaturationOutDataTypeStr=Inherit: Same as second input  DerivativeSourceVariant=Disabled  PreIntVariant=InternalPreInt
  PID Controller4 : slpidlib/PID Controller  Controller=P  Form=Parallel  TimeDomain=Discrete-time  UseExternalTs=off  SampleTime=-1  IntegratorMethod=Forward Euler  FilterMethod=Forward Euler  ControllerParametersSource=internal  P=4  I=1  UseKiTs=off  D=0  UseExternalDerivativeSource=off  N=100  UseFilter=on  TunerSelectOption=Transfer Function Based (PID Tuner App)  InitialConditionSource=internal  InitialConditionForIntegrator=0  InitialConditionForFilter=0  DifferentiatorICPrevScaledInput=0  ExternalReset=none  TrackingMode=off  Kt=1  LimitOutput=off  SatLimitsSource=internal  UpperSaturationLimit=inf  LowerSaturationLimit=-inf  LinearizeAsGain=on  AntiWindupMode=none  Kb=1  LimitIntegrator=off  UpperIntegratorSaturationLimit=inf  LowerIntegratorSaturationLimit=-inf  POutMin=[]  POutMax=[]  IOutMin=[]  IOutMax=[]  DOutMin=[]  DOutMax=[]  NOutMin=[]  NOutMax=[]  SumOutMin=[]  SumOutMax=[]  SaturationOutMin=[]  SaturationOutMax=[]  PParamMin=[]  PParamMax=[]  IParamMin=[]  IParamMax=[]  DParamMin=[]  DParamMax=[]  NParamMin=[]  NParamMax=[]  KbParamMin=[]  KbParamMax=[]  KtParamMin=[]  KtParamMax=[]  KbOutMin=[]  KbOutMax=[]  KtOutMin=[]  KtOutMax=[]  IntegratorOutMin=[]  IntegratorOutMax=[]  FilterOutMin=[]  FilterOutMax=[]  SumI1OutMin=[]  SumI1OutMax=[]  SumI2OutMin=[]  SumI2OutMax=[]  SumI3OutMin=[]  SumI3OutMax=[]  SumI4OutMin=[]  SumI4OutMax=[]  SumDOutMin=[]  SumDOutMax=[]  DifferentiatorOutMin=[]  DifferentiatorOutMax=[]  FilterDiffOutCoefMin=[]  FilterDiffOutCoefMax=[]  ReciprocalOutMin=[]  ReciprocalOutMax=[]  SumDenOutMin=[]  SumDenOutMax=[]  SumNumOutMin=[]  SumNumOutMax=[]  DivideOutMin=[]  DivideOutMax=[]  UdiffTsProdOutMin=[]  UdiffTsProdOutMax=[]  NTsProdOutMin=[]  NTsProdOutMax=[]  UintegralTsProdOutMin=[]  UintegralTsProdOutMax=[]  UngainTsProdOutMin=[]  UngainTsProdOutMax=[]  ClampingZeroOutDataTypeStr=Inherit: Inherit via back propagation  ClampingZeroOutMin=[]  ClampingZeroOutMax=[]  FilterDenConstantOutDataTypeStr=Inherit: Inherit via back propagation  FilterDenConstantOutMin=[]  FilterDenConstantOutMax=[]  PCopyOutDataTypeStr=Inherit: Inherit via back propagation  PCopyOutMin=[]  PCopyOutMax=[]  NCopyOutDataTypeStr=Inherit: Inherit via back propagation  NCopyOutMin=[]  NCopyOutMax=[]  IntegratorContinuousStateAttributes=''  IntegratorStateMustResolveToSignalObject=off  IntegratorRTWStateStorageClass=Auto  FilterContinuousStateAttributes=''  FilterStateMustResolveToSignalObject=off  FilterRTWStateStorageClass=Auto  ParallelPVariant=InternalParameters  IdealPVariant=Disabled  IVariant=Disabled  DVariant=Disabled  IntegratorVariant=Disabled  SatVariant=Disabled  AWVariant=Disabled  PCopyVariant=Disabled  TRVariant=Disabled  FdbkBlocksVariant=Forward  IdealPFdbkVariant=Disabled  SatFdbkVariant=Disabled  DerivativeFilterVariant=Disabled  NVariant=Disabled  NCopyVariant=Disabled_SignalSpec  FilterICVariant=Disabled  IntegratorICVariant=Disabled  ExternalResetVariant=Disabled  TRSumVariant=Passthrough  SumFdbkVariant=Disabled  SumVariant=Passthrough_P  TsampFilterVariant=InternalTs  TsampNgainVariant=Passthrough  TsampIntegralVariant=Disabled_SignalSpec  ExternalSaturationOutDataTypeStr=Inherit: Same as second input  DerivativeSourceVariant=Disabled  PreIntVariant=InternalPreInt
  PID Controller5 : slpidlib/PID Controller  Controller=P  Form=Parallel  TimeDomain=Discrete-time  UseExternalTs=off  SampleTime=-1  IntegratorMethod=Forward Euler  FilterMethod=Forward Euler  ControllerParametersSource=internal  P=2  I=1  UseKiTs=off  D=0  UseExternalDerivativeSource=off  N=100  UseFilter=on  TunerSelectOption=Transfer Function Based (PID Tuner App)  InitialConditionSource=internal  InitialConditionForIntegrator=0  InitialConditionForFilter=0  DifferentiatorICPrevScaledInput=0  ExternalReset=none  TrackingMode=off  Kt=1  LimitOutput=on  SatLimitsSource=internal  UpperSaturationLimit=50*pi/180  LowerSaturationLimit=-50*pi/180  LinearizeAsGain=on  AntiWindupMode=none  Kb=1  LimitIntegrator=off  UpperIntegratorSaturationLimit=inf  LowerIntegratorSaturationLimit=-inf  POutMin=[]  POutMax=[]  IOutMin=[]  IOutMax=[]  DOutMin=[]  DOutMax=[]  NOutMin=[]  NOutMax=[]  SumOutMin=[]  SumOutMax=[]  SaturationOutMin=[]  SaturationOutMax=[]  PParamMin=[]  PParamMax=[]  IParamMin=[]  IParamMax=[]  DParamMin=[]  DParamMax=[]  NParamMin=[]  NParamMax=[]  KbParamMin=[]  KbParamMax=[]  KtParamMin=[]  KtParamMax=[]  KbOutMin=[]  KbOutMax=[]  KtOutMin=[]  KtOutMax=[]  IntegratorOutMin=[]  IntegratorOutMax=[]  FilterOutMin=[]  FilterOutMax=[]  SumI1OutMin=[]  SumI1OutMax=[]  SumI2OutMin=[]  SumI2OutMax=[]  SumI3OutMin=[]  SumI3OutMax=[]  SumI4OutMin=[]  SumI4OutMax=[]  SumDOutMin=[]  SumDOutMax=[]  DifferentiatorOutMin=[]  DifferentiatorOutMax=[]  FilterDiffOutCoefMin=[]  FilterDiffOutCoefMax=[]  ReciprocalOutMin=[]  ReciprocalOutMax=[]  SumDenOutMin=[]  SumDenOutMax=[]  SumNumOutMin=[]  SumNumOutMax=[]  DivideOutMin=[]  DivideOutMax=[]  UdiffTsProdOutMin=[]  UdiffTsProdOutMax=[]  NTsProdOutMin=[]  NTsProdOutMax=[]  UintegralTsProdOutMin=[]  UintegralTsProdOutMax=[]  UngainTsProdOutMin=[]  UngainTsProdOutMax=[]  ClampingZeroOutDataTypeStr=Inherit: Inherit via back propagation  ClampingZeroOutMin=[]  ClampingZeroOutMax=[]  FilterDenConstantOutDataTypeStr=Inherit: Inherit via back propagation  FilterDenConstantOutMin=[]  FilterDenConstantOutMax=[]  PCopyOutDataTypeStr=Inherit: Inherit via back propagation  PCopyOutMin=[]  PCopyOutMax=[]  NCopyOutDataTypeStr=Inherit: Inherit via back propagation  NCopyOutMin=[]  NCopyOutMax=[]  IntegratorContinuousStateAttributes=''  IntegratorStateMustResolveToSignalObject=off  IntegratorRTWStateStorageClass=Auto  FilterContinuousStateAttributes=''  FilterStateMustResolveToSignalObject=off  FilterRTWStateStorageClass=Auto  ParallelPVariant=InternalParameters  IdealPVariant=Disabled  IVariant=Disabled  DVariant=Disabled  IntegratorVariant=Disabled  SatVariant=Enabled  AWVariant=Disabled  PCopyVariant=Disabled  TRVariant=Disabled  FdbkBlocksVariant=Forward  IdealPFdbkVariant=Disabled  SatFdbkVariant=Disabled  DerivativeFilterVariant=Disabled  NVariant=Disabled  NCopyVariant=Disabled_SignalSpec  FilterICVariant=Disabled  IntegratorICVariant=Disabled  ExternalResetVariant=Disabled  TRSumVariant=Passthrough  SumFdbkVariant=Disabled  SumVariant=Passthrough_P  TsampFilterVariant=InternalTs  TsampNgainVariant=Passthrough  TsampIntegralVariant=Disabled_SignalSpec  ExternalSaturationOutDataTypeStr=Inherit: Same as second input  DerivativeSourceVariant=Disabled  PreIntVariant=InternalPreInt
  Rate Limiter1 : RateLimiter  RisingSlewLimit=40*pi/180  FallingSlewLimit=-40*pi/180  SampleTimeMode=inherited
  Rate Limiter2 : RateLimiter  RisingSlewLimit=40*pi/180  FallingSlewLimit=-40*pi/180  SampleTimeMode=inherited
  Saturation : Saturate  UpperLimit=20*pi/180  LowerLimit=-20*pi/180
  Saturation1 : Saturate  UpperLimit=20*pi/180  LowerLimit=-20*pi/180
  Sum{,1..5} (6 alike) : Sum  Inputs=|+-
  tau_Yaw : Outport
  tau_Pitch : Outport  Port=2
  tau_Roll : Outport  Port=3
  wires:
  PID Controller/1 -> tau_Yaw/1
  Sum/1 -> PID Controller1/1
  Ang rate/1 -> Demux/1
  Demux/2 -> Sum/2
  PID Controller1/1 -> tau_Pitch/1
  Sum1/1 -> PID Controller2/1
  Demux/1 -> Sum1/2
  PID Controller2/1 -> tau_Roll/1
  Sum2/1 -> PID Controller3/1
  Sum3/1 -> PID Controller4/1
  ypr/1 -> Demux2/1
  Demux2/2 -> Sum2/2
  Demux2/3 -> Sum3/2
  Sum4/1 -> PID Controller/1
  Demux/3 -> Sum4/2
  Demux2/1 -> Sum5/2
  Sum5/1 -> Calculate minimum Turn/1(In1)
  Calculate minimum Turn/1(Out1) -> PID Controller5/1
  des_roll/1 -> Rate Limiter1/1
  Rate Limiter1/1 -> Saturation/1
  Rate Limiter2/1 -> Saturation1/1
  des_yaw/1 -> Sum5/1
  Saturation/1 -> Sum3/1
  PID Controller3/1 -> Sum/1
  Saturation1/1 -> Sum2/1
  des_pitch/1 -> Rate Limiter2/1
  PID Controller4/1 -> Sum1/1
  PID Controller5/1 -> Sum4/1
